simulink model "ex4_18"  (R2023b)
settings: Solver=VariableStepAuto  StartTime=0.0  StopTime=10.0  RelTol=1e-3
model workspace (MAT data in the model file):
  Fg = Simulink.Parameter
  Fg.Value = 10
  Fg.DataType = 'auto'
  Fg.DocUnits = 'N'
  Fg.Complexity = 'real'
  Fg.Dimensions = [1 1]
  c = Simulink.Parameter
  c.Value = 0.1
  c.DataType = 'auto'
  c.DocUnits = 'm/N'
  c.Complexity = 'real'
  c.Dimensions = [1 1]
  f = Simulink.Parameter
  f.Value = 3
  f.DataType = 'auto'
  f.DocUnits = 'N*1/m*s*s'
  f.Complexity = 'real'
  f.Dimensions = [1 1]
  m = Simulink.Parameter
  m.Value = 10
  m.DataType = 'auto'
  m.DocUnits = 'kg'
  m.Complexity = 'real'
  m.Dimensions = [1 1]
settings Model: Creator=morten  LastModifiedBy=morten

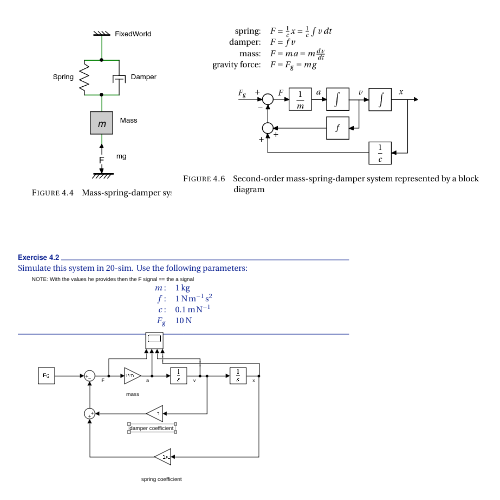
[thumbnail: Simulink's stored preview of the top-level diagram]
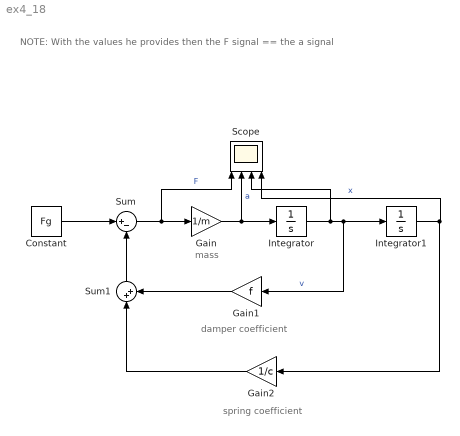
== system ex4_18 ==
  note: NOTE: With the values he provides then the F signal == the a signal
  note: mass
  note: damper coefficient
  note: spring coefficient
  Constant : Constant  Value=Fg
  Gain : Gain  Gain=1/m
  Gain1 : Gain  Gain=f
  Gain2 : Gain  Gain=1/c
  Integrator : Integrator
  Integrator1 : Integrator
  Scope : Scope  NumInputPorts=4
  Sum : Sum  Inputs=|+-
  Sum1 : Sum  Inputs=|++
  wires:
  Constant/1 -> Sum/1
  Integrator/1 -> Scope/3, Gain1/1, Integrator1/1  "v"
  Gain1/1 -> Sum1/2
  Sum1/1 -> Sum/2
  Integrator1/1 -> Gain2/1, Scope/4  "x"
  Sum/1 -> Gain/1, Scope/1  "F"
  Gain/1 -> Scope/2, Integrator/1  "a"
  Gain2/1 -> Sum1/1
